simulink model "MasaEjemplo1"  (Simulink 5.0)
settings: Solver=ode45  StartTime=0.0  StopTime=5  RelTol=1e-3
values from neighbouring files (symbols this model uses):
  B = 20    [MasaEjemplo1_valores.m]    (also in VariablesMotorCD.m = 0.01)
  K = 160    [MasaEjemplo1_valores.m]
  M = 0.4    [MasaEjemplo1_valores.m]
settings Model: LastModifiedBy=gaby

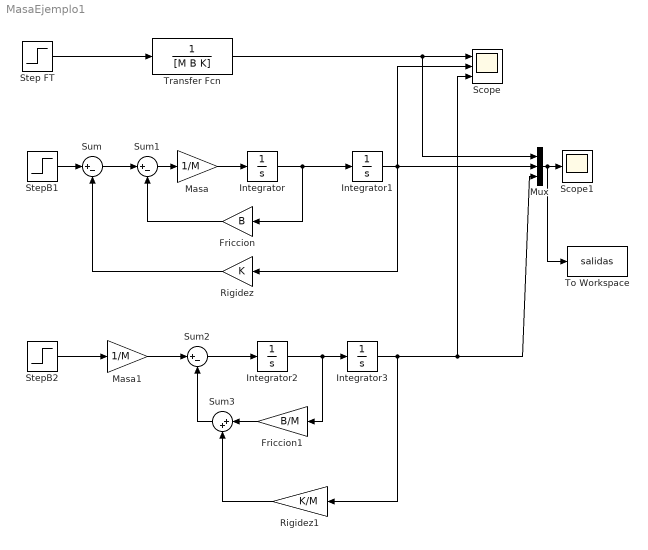
== system MasaEjemplo1 ==
  Friccion : Gain  Orientation=left  Gain=B  SaturateOnIntegerOverflow=on
  Friccion1 : Gain  Orientation=left  Gain=B/M  SaturateOnIntegerOverflow=on
  Integrator{,1..3} (4 alike) : Integrator
  Masa : Gain  Gain=1/M  SaturateOnIntegerOverflow=on
  Masa1 : Gain  Gain=1/M  SaturateOnIntegerOverflow=on
  Mux : Mux  Inputs=3
  Rigidez : Gain  Orientation=left  Gain=K  SaturateOnIntegerOverflow=on
  Rigidez1 : Gain  Orientation=left  Gain=K/M  SaturateOnIntegerOverflow=on
  Scope : Scope  NumInputPorts=3
      settings: YMin=-5~-5~-5  YMax=5~5~5
  Scope1 : Scope
  Step FT : Step  Time=0  SampleTime=0
  StepB1 : Step  Time=0.1  SampleTime=0
  StepB2 : Step  Time=0.2  SampleTime=0
  Sum : Sum  Inputs=|+-  SaturateOnIntegerOverflow=on
  Sum1 : Sum  Inputs=|+-  SaturateOnIntegerOverflow=on
  Sum2 : Sum  Inputs=|+-  SaturateOnIntegerOverflow=on
  Sum3 : Sum  Orientation=left  Inputs=|++  SaturateOnIntegerOverflow=on
  To Workspace : ToWorkspace  VariableName=salidas  SampleTime=-1  SaveFormat=Array
  Transfer Fcn : TransferFcn  Denominator=[M B K]
  wires:
  Step FT/1 -> Transfer Fcn/1
  Transfer Fcn/1 -> Scope/1, Mux/1
  Masa/1 -> Integrator/1
  Integrator/1 -> Integrator1/1, Friccion/1
  Integrator1/1 -> Rigidez/1, Scope/2, Mux/2
  StepB1/1 -> Sum/1
  Sum/1 -> Sum1/1
  Sum1/1 -> Masa/1
  Friccion/1 -> Sum1/2
  Rigidez/1 -> Sum/2
  StepB2/1 -> Masa1/1
  Masa1/1 -> Sum2/1
  Sum2/1 -> Integrator2/1
  Integrator2/1 -> Integrator3/1, Friccion1/1
  Integrator3/1 -> Rigidez1/1, Scope/3, Mux/3
  Friccion1/1 -> Sum3/1
  Rigidez1/1 -> Sum3/2
  Sum3/1 -> Sum2/2
  Mux/1 -> Scope1/1, To Workspace/1
